simulink model "Test7"  (R2021a)
settings: Solver=FixedStepDiscrete  StartTime=0.0  StopTime=tsim  FixedStep=Ts  RelTol=1e-3  EnableMultiTasking=on
InitFcn:
  | Fs = 2048; Ts = 1/Fs;tsim = inf;
undefined symbols (not defined in the file or in its folder): DiscIntNeverNeededParam
libraries: sperte_lib x26, simulink x5, Quintic_Polynomial_Trajectory_Library x3, raspberrypiCommlib x2
(part 1 of 2)
settings Model: SimulationMode=external  Creator=20174295  LastModifiedBy=20212540
settings SolverCC: AlgebraicLoopSolver=TrustRegion  PositivePriorityOrder=on
settings DataIOCC: SaveOutput=off  DSMLogging=off  SaveTime=off  ReturnWorkspaceOutputs=off
settings OptimizationCC: EnhancedBackFolding=on  PassReuseOutputArgsThreshold=0  MaxStackSize=64  OptimizeBlockOrder=speed  DifferentSizesBufferReuse=on  OptimizationCustomize=off
settings DebuggingCC: InheritedTsInSrcMsg=none  ParameterTunabilityLossMsg=error  SFMachineParentedDataDiag=warning
settings HardwareCC: ProdBitPerPointer=32  ProdBitPerSizeT=32  ProdBitPerPtrDiffT=32  ProdLargestAtomicInteger=Long  ProdLargestAtomicFloat=Double  ProdWordSize=32  ProdLongLongMode=on  ProdHWDeviceType=ARM Compatible->ARM Cortex  UseEmbeddedCoderFeatures=off
settings RTWCC: SystemTargetFile=ert.tlc  HardwareBoard=Raspberry Pi  TLCOptions="-aInlineSetEventsForThisBaseRateFcn=TLC_FALSE -aSuppressMultiTaskScheduler=TLC_FALSE  -aRateBasedStepFcn=0"  TemplateMakefile=ert_default_tmf  PostCodeGenCommand="if (~verLessThan(\"matlab\", \"9.11\")) codertarget.postCodeGenHookCommand(h);  SPERTE_postGenFunc(modelName, buildInfo); else; SPERTE_postGenFunc(h, buildInfo); end"  Toolchain=GNU GCC Embedded Linux  BuildConfiguration=Faster Runs
settings CodeAppCC: ForceParamTrailComments=on  OperatorAnnotations=on
settings ERTTargetCC: ERTCustomFileBanners=off  SupportContinuousTime=on  SupportNonInlinedSFcns=on  RemoveResetFunc=off  SupportVariableSizeSignals=on  ModelStepFunctionPrototypeControlCompliant=off  ExtMode=on  ExtModeStaticAlloc=on  ExtModeMexArgs='10.55.0.1' 0 17726  ERTSrcFileBannerTemplate=codertarget_code_template.cgt  ERTHdrFileBannerTemplate=codertarget_code_template.cgt  ERTDataSrcFileTemplate=codertarget_code_template.cgt  ERTDataHdrFileTemplate=codertarget_code_template.cgt

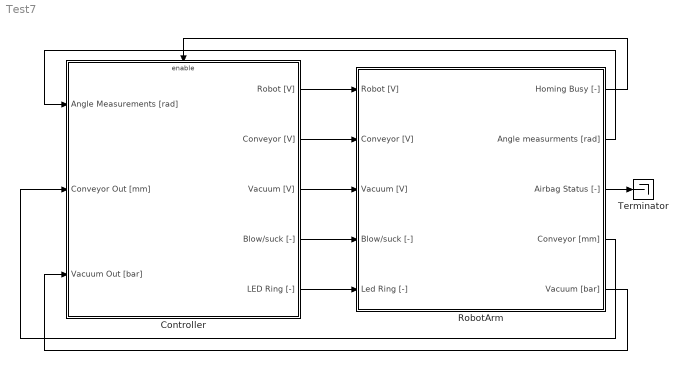
== system Test7 ==
  Controller : Subsystem
  RobotArm : Subsystem
      mask help:
      | Robot Arm
      | Hardware: Brom Mechatronica
      | Software: Victor Dolk, Quinten Swaan, Hugo Thelosen
      mask Display:
      | image(imread('picture_robot.jpg'))
      | color('red');port_label('output', 1, 'Homing Busy [-]')
      | port_label('output', 2, 'Angle Measurements [rad]')
      | port_label('output', 3, 'Airbag Status [-]')
      | port_label('input', 1, 'Input Robot [V]')
      | port_label('output', 4, 'Conveyor Belt [mm]')
      | port_label('output', 5, 'Vacuum Sensor [bar]')
      | port_label('input',2,'Input Conv [V]' )
      | port_label('input',3,'Input Vac [V]' )
      | port_label('input',4,'IO Vac [-]' )
      | port_label('input',5,'LED-Ring [-]' )
  Terminator : Terminator
  wires:
  RobotArm/4(Conveyor [mm]) -> Controller/2(Conveyor Out [mm])
  Controller/5(LED Ring [-]) -> RobotArm/5(Led Ring [-])
  Controller/1(Robot [V]) -> RobotArm/1(Robot [V])
  Controller/4(Blow/suck [-]) -> RobotArm/4(Blow/suck [-])
  RobotArm/1(Homing Busy [-]) -> Controller/Enable
  Controller/3("Vacuum [V] ") -> RobotArm/3(Vacuum [V])
  Controller/2("Conveyor [V] ") -> RobotArm/2(Conveyor [V])
  RobotArm/5(Vacuum [bar]) -> Controller/3(Vacuum Out [bar])
  RobotArm/3(Airbag Status [-]) -> Terminator/1
  RobotArm/2(Angle measurments [rad]) -> Controller/1(Angle Measurements [rad])

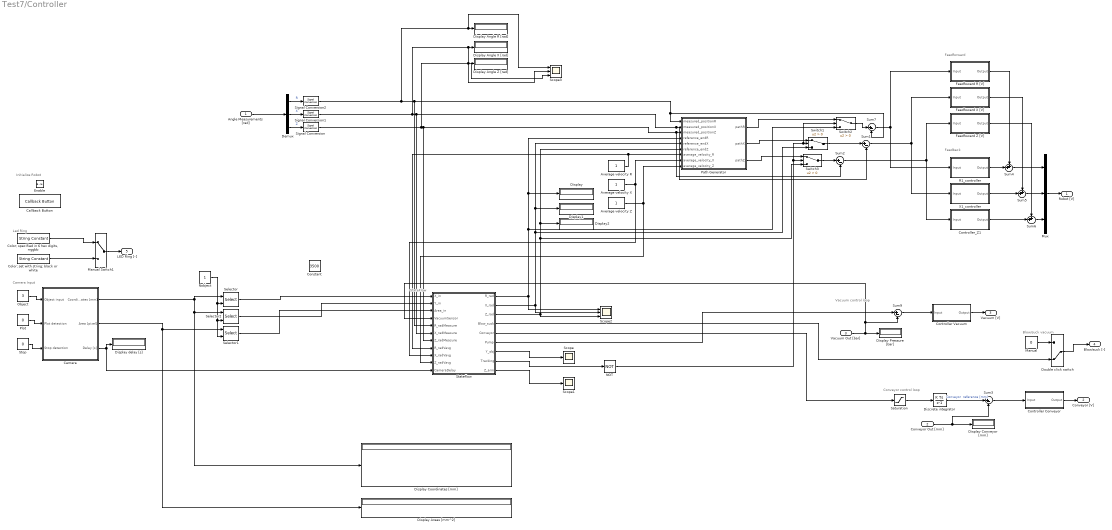
== system Test7/Controller ==
  note: Feedforward
  note: StateFlow
  note: Camera Input
  note: Vacuum control loop
  note: Conveyor control loop
  note: Blow/suck vacuum
  note: Led Ring
  note: Feedback
  note: Initialize Robot
  Angle Measurements [rad] : Inport
  Conveyor Out [mm] : Inport  Port=2
  Vacuum Out [bar] : Inport  Port=3
  "Enable " : EnablePort
  Average velocity R : Constant
  Average velocity X : Constant
  Average velocity Z : Constant
  Callback Button : CallbackButton  ButtonText=INITIALIZE MODEL
      settings: ClickFcn=|
      | robot_number = input('What is your Robot number?: ');
      | file_name_simulink = get_param(bdroot, 'Name');
      | load('calibration_matrix.mat');
      | [camera_calibration_x_pixels,camera_calibration_y_pixels,camera_calibration_pixels_per_mm,camera_calibration_ROI,robot_calibration_r,robot_calibration_x, robot_calibration_z] = Calibrate_Robot_Settings(robot_number,calibration)
      | 
      | set_param(file_name_simulink+"/RobotArm/Supervisor/set_robot_calibration_r",'Value',num2str(robot_calibration_r));
      | set_param(file_name_simulink+"/RobotArm/Supervisor/set_robot_calibration_x",'Value',num2str(robot_calibration_x));
      | set_param(file_name_simulink+"/RobotArm/Supervisor/set_robot_calibration_z",'Value',num2str(robot_calibration_z));
      | 
      | clear calibration
      | msgbox('Successfully initialized the model.');
  Camera : Subsystem
  Color; set with string; black or white : StringConstant  String='white'
  "Color; specified in 6 hex digits, rrggbb" : StringConstant  String='FF0000'
  Constant : Constant  Value=3500
  Controller Conveyor : Subsystem
  Controller Vacuum : Subsystem
  Controller_Z1 : Subsystem
  Demux : Demux  Outputs=3
  Discrete integrator : DiscreteIntegrator  SampleTime=-1  ICPrevOutput=DiscIntNeverNeededParam  ICPrevScaledInput=DiscIntNeverNeededParam
  Display : Display
  Display Angle R [rad] : Display
  Display Angle X [rad] : Display
  Display Angle Z [rad] : Display
  Display Areas [mm^2] : Display
  Display Conveyor [mm] : Display
  Display Coordinates [mm] : Display
  Display Pressure [bar] : Display
  Display delay [s] : Display
  Display1 : Display
  Display2 : Display
  Double click switch : ManualSwitch  CurrentSetting=0
  Feedfoward R [V] : Subsystem
  Feedfoward X [V] : Subsystem
  Feedfoward Z [V] : Subsystem
  Manual : Constant  Value=0
  Manual Switch1 : ManualSwitch
  Mux : Mux  Inputs=3
  NOT : Logic  Operator=NOT  IconShape=distinctive  AllPortsSameDT=off  OutDataTypeStr=boolean
  Nobject : Constant
  Object : Constant  Value=3
  Path Generator : Subsystem
  Plot : Constant  Value=0
  R1_controller : Subsystem
  "Saturation " : Saturate  UpperLimit=100  LowerLimit=-100
  Scope : Scope
  Scope1 : Scope
  Scope2 : Scope  NumInputPorts=3
  Scope3 : Scope  NumInputPorts=3
  Selector : Selector  NumberOfDimensions=2  InputPortWidth=3  IndexOptions=Index vector (dialog),Index vector (port)  Indices=1,1  OutputSizes=1,1
  Selector1 : Selector  InputPortWidth=3  IndexOptions=Index vector (port)  Indices=[1 3]  OutputSizes=1
  Selector2 : Selector  NumberOfDimensions=2  InputPortWidth=3  IndexOptions=Index vector (dialog),Index vector (port)  Indices=2,1  OutputSizes=1,1
  Signal Conversion : SignalConversion  OverrideOpt=off
  Signal Conversion1 : SignalConversion  OverrideOpt=off
  Signal Conversion2 : SignalConversion  OverrideOpt=off
  "Stateflow " : Stateflow chart  TreatAsAtomicUnit=on
  Stop : Constant  Value=0
  Sum1 : Sum  Inputs=|+-  InputSameDT=on  SaturateOnIntegerOverflow=on  OutDataTypeStr=Inherit: Same as first input
  Sum2 : Sum  Inputs=|+-  InputSameDT=on  SaturateOnIntegerOverflow=on  OutDataTypeStr=Inherit: Same as first input
  Sum3 : Sum  Inputs=|+-
  Sum4 : Sum  Inputs=++|  InputSameDT=on  SaturateOnIntegerOverflow=on  OutDataTypeStr=Inherit: Same as first input
  Sum5 : Sum  Inputs=++|  InputSameDT=on  SaturateOnIntegerOverflow=on  OutDataTypeStr=Inherit: Same as first input
  Sum6 : Sum  Inputs=++|  InputSameDT=on  SaturateOnIntegerOverflow=on  OutDataTypeStr=Inherit: Same as first input
  Sum7 : Sum  Inputs=|+-  InputSameDT=on  SaturateOnIntegerOverflow=on  OutDataTypeStr=Inherit: Same as first input
  Sum9 : Sum  Inputs=|+-
  Switch1 : Switch  Criteria=u2 > Threshold
  Switch2 : Switch  Criteria=u2 > Threshold
  Switch3 : Switch  Criteria=u2 > Threshold
  X1_controller : Subsystem
  Robot [V] : Outport
  "Conveyor [V] " : Outport  Port=2
  "Vacuum [V] " : Outport  Port=3
  Blow/suck [-] : Outport  Port=4
  LED Ring [-] : Outport  Port=5
  wires:
  Sum5/1 -> Mux/2
  Sum4/1 -> Mux/1
  Demux/3 -> Signal Conversion/1  "Z"
  Signal Conversion1/1 -> "Stateflow "/6(X_radMeasure), Path Generator/2(measured_positionX), Sum1/2, Scope3/2, Display Angle X [rad]/1
  Angle Measurements [rad]/1 -> Demux/1
  Demux/1 -> Signal Conversion2/1  "R"
  Mux/1 -> Robot [V]/1
  Signal Conversion/1 -> "Stateflow "/7(Z_radMeasure), Path Generator/3(measured_positionZ), Sum2/2, Scope3/3, Display Angle Z [rad]/1
  Sum6/1 -> Mux/3
  Demux/2 -> Signal Conversion1/1  "X"
  Signal Conversion2/1 -> "Stateflow "/5(R_radMeasure), Sum7/2, Path Generator/1(measured_positionR), Scope3/1, Display Angle R [rad]/1
  Manual Switch1/1 -> LED Ring [-]/1
  Conveyor Out [mm]/1 -> Sum3/2, Display Conveyor [mm]/1
  Color; set with string; black or white/1 -> Manual Switch1/2
  "Color; specified in 6 hex digits, rrggbb"/1 -> Manual Switch1/1
  Camera/1(Coordinates [mm]) -> Selector/1, Display Coordinates [mm]/1, Selector2/1
  Controller Vacuum/1(Output) -> "Vacuum [V] "/1
  Sum9/1 -> Controller Vacuum/1(Input)
  Vacuum Out [bar]/1 -> Sum9/2, "Stateflow "/4(VacuumSensor), Display Pressure [bar]/1
  Camera/2(Area [pixel]) -> Display Areas [mm^2]/1, Selector1/1
  Camera/3(Delay [s]) -> Display delay [s]/1, "Stateflow "/11(CameraDelay)
  Manual/1 -> Double click switch/1
  Plot/1 -> Camera/2(Plot detection)
  Object/1 -> Camera/1(Object input)
  Stop/1 -> Camera/3(Stop detection)
  Double click switch/1 -> Blow/suck [-]/1
  "Saturation "/1 -> Discrete integrator/1
  Discrete integrator/1 -> Sum3/1  "Conveyor  reference [mm]"
  Sum3/1 -> Controller Conveyor/1(Input)
  Controller Conveyor/1(Output) -> "Conveyor [V] "/1
  Feedfoward R [V]/1(Output) -> Sum4/1
  "Stateflow "/5(Conveyor) -> "Saturation "/1
  "Stateflow "/4(Blow_suck) -> Double click switch/2
  Nobject/1 -> Selector1/2, Selector2/2, Selector/2
  Selector1/1 -> "Stateflow "/3(Area_in)
  Sum7/1 -> R1_controller/1(Input), Feedfoward R [V]/1(Input)
  Sum1/1 -> X1_controller/1(Input), Feedfoward X [V]/1(Input)
  Sum2/1 -> Feedfoward Z [V]/1(Input), Controller_Z1/1(Input)
  Feedfoward X [V]/1(Output) -> Sum5/1
  Feedfoward Z [V]/1(Output) -> Sum6/1
  Average velocity R/1 -> Path Generator/7(average_velocity_R), "Stateflow "/8(R_radVavg)
  Average velocity X/1 -> Path Generator/8(average_velocity_X), "Stateflow "/9(X_radVavg)
  Average velocity Z/1 -> "Stateflow "/10(Z_radVavg), Path Generator/9(average_velocity_Z)
  "Stateflow "/6(Pump) -> Sum9/1
  R1_controller/1(Output) -> Sum4/2
  X1_controller/1(Output) -> Sum5/2
  Controller_Z1/1(Output) -> Sum6/2
  Selector2/1 -> "Stateflow "/2(Y_in)
  Path Generator/2(pathX) -> Switch1/1
  Path Generator/3(pathZ) -> Switch3/1
  "Stateflow "/1(R_rad) -> Scope2/1, Path Generator/4(reference_endR), Display/1, Switch2/3
  "Stateflow "/2(X_rad) -> Scope2/2, Display1/1, Path Generator/5(reference_endX), Switch1/3
  "Stateflow "/3(Z_rad) -> Scope2/3, Display2/1, Path Generator/6(reference_endZ), Switch3/3
  Path Generator/1(pathR) -> Switch2/1
  "Stateflow "/7(Y_obj) -> Scope/1
  Selector/1 -> "Stateflow "/1(X_in)
  Switch2/1 -> Sum7/1
  Switch1/1 -> Sum1/1
  Switch3/1 -> Sum2/1
  NOT/1 -> Switch3/2, Switch2/2, Switch1/2
  "Stateflow "/8(Tracking) -> NOT/1
  "Stateflow "/9(Z_arm) -> Scope1/1

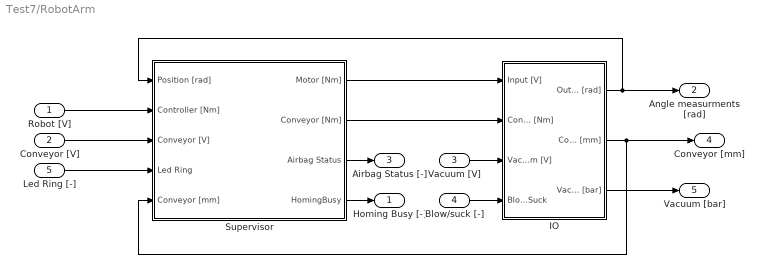
== system Test7/RobotArm ==
  Robot [V] : Inport
  Conveyor [V] : Inport  Port=2
  Vacuum [V] : Inport  Port=3
  Blow/suck [-] : Inport  Port=4
  Led Ring [-] : Inport  Port=5
  IO : Subsystem
  Supervisor : Subsystem
  Homing Busy [-] : Outport
  Angle measurments [rad] : Outport  Port=2
  Airbag Status [-] : Outport  Port=3
  Conveyor [mm] : Outport  Port=4
  Vacuum [bar] : Outport  Port=5
  wires:
  Robot [V]/1 -> Supervisor/2(Controller [Nm])
  IO/1(Output [rad]) -> Supervisor/1(Position [rad]), Angle measurments [rad]/1
  Supervisor/4(HomingBusy) -> Homing Busy [-]/1
  Supervisor/3(Airbag Status) -> Airbag Status [-]/1
  Supervisor/1(Motor [Nm]) -> IO/1(Input [V])
  IO/3(Vacuum [bar]) -> Vacuum [bar]/1
  Conveyor [V]/1 -> Supervisor/3(Conveyor [V])
  Vacuum [V]/1 -> IO/3(Vacuum [V])
  Supervisor/2(Conveyor [Nm]) -> IO/2(Conveyor [Nm])
  Blow/suck [-]/1 -> IO/4(Blow_Suck)
  IO/2(Conveyor [mm]) -> Supervisor/5(Conveyor [mm]), Conveyor [mm]/1
  Led Ring [-]/1 -> Supervisor/4(Led Ring)

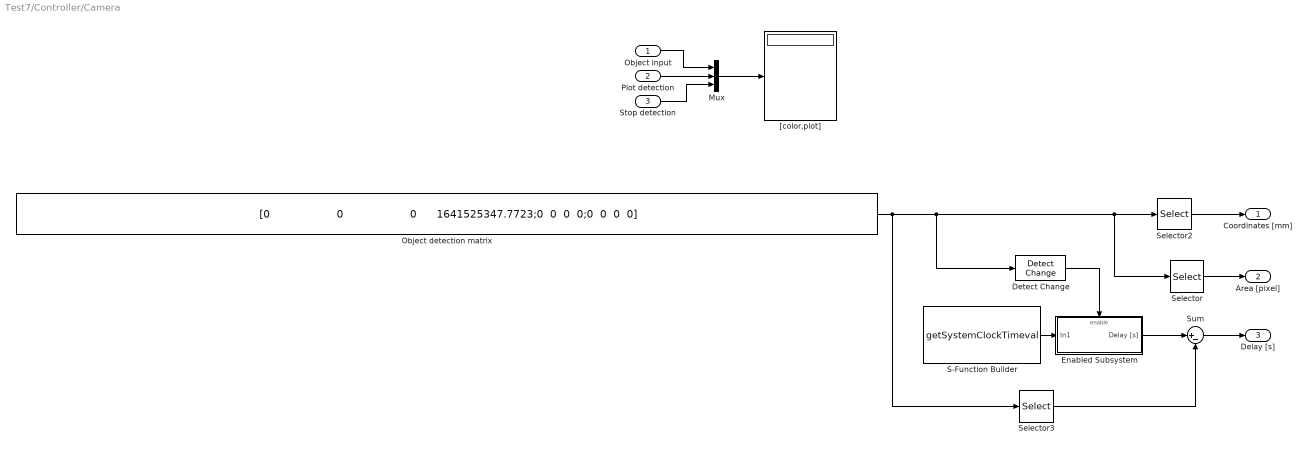
== system Test7/Controller/Camera ==
  Object input : Inport
  Plot detection : Inport  Port=2
  Stop detection : Inport  Port=3
  Detect Change : simulink/Logic and Bit Operations/Detect Change  vinit=0  OutDataTypeStr=boolean
  Enabled Subsystem : Subsystem  TreatAsAtomicUnit=on
  Mux : Mux  Inputs=3
  Object detection matrix : Constant  Value="[0                    0                    0      1641525347.7723;0  0  0  0;0  0  0  0]"  VectorParams1D=off
  S-Function Builder : S-Function  InitFcn=try, set_param(gcb,'FunctionName','getSystemClockTimeval'), end  FunctionName=getSystemClockTimeval  SFunctionModules=getSystemClockTimeval_wrapper  SFunctionDeploymentMode=off  EnableBusSupport=off  mask(S-Function Builder){}
      mask help: Simulink:masks:SFunctionBuilder_MD
      mask init:
      | val = [[.9  0.75 0.75 1 1 .9 .9 1]',[1 1 0.75 0.75 .9 .9 1 .9]'];try , sys = get_param(gcb,'SfunBuilderFcnName');if isempty(sys), sys = get_param(gcb,'FunctionName'); end,catch, sys = get_param(gcb,'FunctionName'); end
      settings: CopyFcn=set_param(gcbh,'LinkStatus','none')  PreSaveFcn=try, set_param(gcb,'FunctionName','getSystemClockTimeval'), end  OpenFcn=sfunctionwizard(gcbh)
      mask Display: plot(val(:,1),val(:,2)),disp(sys),port_label('output',1,'y2')
  Selector : Selector  NumberOfDimensions=2  InputPortWidth=3  IndexOptions=Index vector (dialog),Index vector (dialog)  Indices=[3],[1:3]  OutputSizes=1,1
  Selector2 : Selector  NumberOfDimensions=2  InputPortWidth=3  IndexOptions=Index vector (dialog),Index vector (dialog)  Indices=[1:2],[1:3]  OutputSizes=1,1
  Selector3 : Selector  NumberOfDimensions=2  InputPortWidth=3  IndexOptions=Index vector (dialog),Index vector (dialog)  Indices=1,4  OutputSizes=1,1
  Sum : Sum  Inputs=|+-
  "[color,plot]" : Display
  Coordinates [mm] : Outport
  Area [pixel] : Outport  Port=2
  Delay [s] : Outport  Port=3
  wires:
  Object input/1 -> Mux/1
  Plot detection/1 -> Mux/2
  Mux/1 -> "[color,plot]"/1
  Stop detection/1 -> Mux/3
  Selector2/1 -> Coordinates [mm]/1
  Object detection matrix/1 -> Selector3/1, Detect Change/1, Selector/1, Selector2/1
  Detect Change/1 -> Enabled Subsystem/Enable
  S-Function Builder/1 -> Enabled Subsystem/1(In1)
  Enabled Subsystem/1(Delay [s]) -> Sum/1
  Sum/1 -> Delay [s]/1
  Selector3/1 -> Sum/2
  Selector/1 -> Area [pixel]/1

== system Test7/Controller/Controller Conveyor ==
  Input : Inport
  Dct1lowpass : sperte_lib/Dct1lowpass  f_den=30
      settings: SourceProductName=SPERTE project library
  Dctintegrator3 : S-Function  FunctionName=dweakint  Parameters=f_num, 0.001  SFunctionDeploymentMode=off  EnableBusSupport=off  mask(dctools){f_num=0}
      mask prompts: f_num "Zero [Hz]"
      mask help: This block implements a discrete time weak integrator filter.
      mask Display: disp('DCT integrator')
  Dctleadlag : sperte_lib/Dctleadlag  f_num=3  f_den=20
      settings: SourceProductName=SPERTE project library
  Gain1 : Gain  Gain=10*2.5/500
  Output : Outport
  wires:
  Input/1 -> Gain1/1
  Dctintegrator3/1 -> Dct1lowpass/1
  Dctleadlag/1 -> Output/1
  Gain1/1 -> Dctintegrator3/1
  Dct1lowpass/1 -> Dctleadlag/1

== system Test7/Controller/Controller Vacuum ==
  Input : Inport
  Gain1 : Gain  Gain=-10
  Output : Outport
  wires:
  Input/1 -> Gain1/1
  Gain1/1 -> Output/1

== system Test7/Controller/Controller_Z1 ==
  Input : Inport
  Dct1lowpass1 : sperte_lib/Dct1lowpass  f_den=200
      settings: SourceProductName=SPERTE project library
  Dctintegrator2 : S-Function  FunctionName=dweakint  Parameters=f_num, 0.001  SFunctionDeploymentMode=off  EnableBusSupport=off  mask(dctools){f_num=1.7}
      mask prompts: f_num "Zero [Hz]"
      mask help: This block implements a discrete time weak integrator filter.
      mask Display: disp('DCT integrator')
  Dctleadlag3 : S-Function  FunctionName=dleadlag  Parameters=f_num, f_den, 0.001  SFunctionDeploymentMode=off  EnableBusSupport=off  mask(dctools){f_num=7, f_den=75}
      mask prompts: f_num "Zero [Hz]"; f_den "Pole [Hz]"
      mask help: This block implements a discrete time leadlag filter.
      mask Display: disp('DCT leadlag')
  Gain2 : Gain  Gain=25
  Output : Outport
  wires:
  Input/1 -> Gain2/1
  Dctintegrator2/1 -> Dctleadlag3/1
  Gain2/1 -> Dctintegrator2/1
  Dctleadlag3/1 -> Dct1lowpass1/1
  Dct1lowpass1/1 -> Output/1

== system Test7/Controller/Feedfoward R [V] ==
  Input : Inport
  Derivative : Derivative
  Derivative1 : Derivative
  Gain1 : Gain  Gain=0
  Gain2 : Gain  Gain=0
  Inertia compensation : Gain  Gain=0
  Sign : Signum
  Sum : Sum  Inputs=+++
  Output : Outport
  wires:
  Input/1 -> Derivative/1
  Derivative/1 -> Sign/1, Gain1/1, Derivative1/1
  Sum/1 -> Output/1
  Gain2/1 -> Sum/1
  Gain1/1 -> Sum/2
  Inertia compensation/1 -> Sum/3
  Derivative1/1 -> Inertia compensation/1
  Sign/1 -> Gain2/1

== system Test7/Controller/Feedfoward X [V] ==
  Input : Inport
  Derivative : Derivative
  Derivative1 : Derivative
  Gain1 : Gain  Gain=0
  Gain2 : Gain  Gain=0
  Inertia compensation : Gain  Gain=0
  Sign : Signum
  Sum : Sum  Inputs=+++
  Output : Outport
  wires:
  Sign/1 -> Gain2/1
  Sum/1 -> Output/1
  Gain1/1 -> Sum/2
  Gain2/1 -> Sum/1
  Derivative1/1 -> Inertia compensation/1
  Inertia compensation/1 -> Sum/3
  Derivative/1 -> Sign/1, Gain1/1, Derivative1/1
  Input/1 -> Derivative/1

== system Test7/Controller/Feedfoward Z [V] ==
  Input : Inport
  Derivative : Derivative
  Derivative1 : Derivative
  Gain1 : Gain  Gain=0
  Gain2 : Gain  Gain=0
  Inertia compensation : Gain  Gain=0
  Sign : Signum
  Sum : Sum  Inputs=+++
  Output : Outport
  wires:
  Sign/1 -> Gain2/1
  Sum/1 -> Output/1
  Gain1/1 -> Sum/2
  Gain2/1 -> Sum/1
  Derivative1/1 -> Inertia compensation/1
  Inertia compensation/1 -> Sum/3
  Derivative/1 -> Sign/1, Gain1/1, Derivative1/1
  Input/1 -> Derivative/1

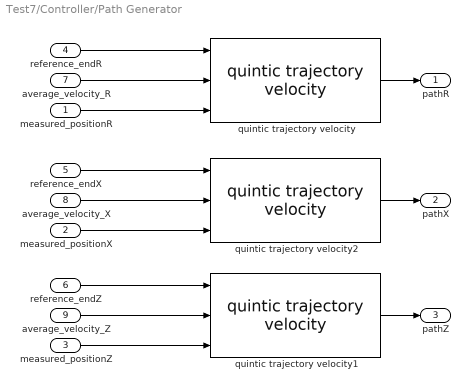
== system Test7/Controller/Path Generator ==
  measured_positionR : Inport
  measured_positionX : Inport  Port=2
  measured_positionZ : Inport  Port=3
  reference_endR : Inport  Port=4
  reference_endX : Inport  Port=5
  reference_endZ : Inport  Port=6
  average_velocity_R : Inport  Port=7
  average_velocity_X : Inport  Port=8
  average_velocity_Z : Inport  Port=9
  quintic trajectory velocity : Quintic_Polynomial_Trajectory_Library/quintic trajectory velocity  SystemSampleTime=-1  VariantActivationTime=update diagram  Latency=0  AutoFrameSizeCalculation=off
      settings: SourceProductName=Robotarm library
  quintic trajectory velocity1 : Quintic_Polynomial_Trajectory_Library/quintic trajectory velocity  SystemSampleTime=-1  VariantActivationTime=update diagram  Latency=0  AutoFrameSizeCalculation=off
      settings: SourceProductName=Robotarm library
  quintic trajectory velocity2 : Quintic_Polynomial_Trajectory_Library/quintic trajectory velocity  SystemSampleTime=-1  VariantActivationTime=update diagram  Latency=0  AutoFrameSizeCalculation=off
      settings: SourceProductName=Robotarm library
  pathR : Outport
  pathX : Outport  Port=2
  pathZ : Outport  Port=3
  wires:
  reference_endR/1 -> quintic trajectory velocity/1
  measured_positionR/1 -> quintic trajectory velocity/3
  average_velocity_R/1 -> quintic trajectory velocity/2
  average_velocity_X/1 -> quintic trajectory velocity2/2
  average_velocity_Z/1 -> quintic trajectory velocity1/2
  measured_positionX/1 -> quintic trajectory velocity2/3
  measured_positionZ/1 -> quintic trajectory velocity1/3
  reference_endX/1 -> quintic trajectory velocity2/1
  reference_endZ/1 -> quintic trajectory velocity1/1
  quintic trajectory velocity/1 -> pathR/1
  quintic trajectory velocity2/1 -> pathX/1
  quintic trajectory velocity1/1 -> pathZ/1

== system Test7/Controller/R1_controller ==
  Input : Inport
  Dct1lowpass1 : sperte_lib/Dct1lowpass  f_den=100
      settings: SourceProductName=SPERTE project library
  Dctintegrator2 : S-Function  FunctionName=dweakint  Parameters=f_num, 0.001  SFunctionDeploymentMode=off  EnableBusSupport=off  mask(dctools){f_num=1.35}
      mask prompts: f_num "Zero [Hz]"
      mask help: This block implements a discrete time weak integrator filter.
      mask Display: disp('DCT integrator')
  Dctleadlag3 : S-Function  FunctionName=dleadlag  Parameters=f_num, f_den, 0.001  SFunctionDeploymentMode=off  EnableBusSupport=off  mask(dctools){f_num=8, f_den=75}
      mask prompts: f_num "Zero [Hz]"; f_den "Pole [Hz]"
      mask help: This block implements a discrete time leadlag filter.
      mask Display: disp('DCT leadlag')
  Gain1 : Gain  Gain=40
  Output : Outport
  wires:
  Gain1/1 -> Dctintegrator2/1
  Dctintegrator2/1 -> Dctleadlag3/1
  Input/1 -> Gain1/1
  Dctleadlag3/1 -> Dct1lowpass1/1
  Dct1lowpass1/1 -> Output/1

== system Test7/Controller/X1_controller ==
  Input : Inport
  Dct1lowpass1 : sperte_lib/Dct1lowpass  f_den=200
      settings: SourceProductName=SPERTE project library
  Dctintegrator2 : S-Function  FunctionName=dweakint  Parameters=f_num, 0.001  SFunctionDeploymentMode=off  EnableBusSupport=off  mask(dctools){f_num=2}
      mask prompts: f_num "Zero [Hz]"
      mask help: This block implements a discrete time weak integrator filter.
      mask Display: disp('DCT integrator')
  Dctleadlag3 : S-Function  FunctionName=dleadlag  Parameters=f_num, f_den, 0.001  SFunctionDeploymentMode=off  EnableBusSupport=off  mask(dctools){f_num=10, f_den=70}
      mask prompts: f_num "Zero [Hz]"; f_den "Pole [Hz]"
      mask help: This block implements a discrete time leadlag filter.
      mask Display: disp('DCT leadlag')
  Gain2 : Gain  Gain=17
  Output : Outport
  wires:
  Input/1 -> Gain2/1
  Dctintegrator2/1 -> Dctleadlag3/1
  Gain2/1 -> Dctintegrator2/1
  Dctleadlag3/1 -> Dct1lowpass1/1
  Dct1lowpass1/1 -> Output/1

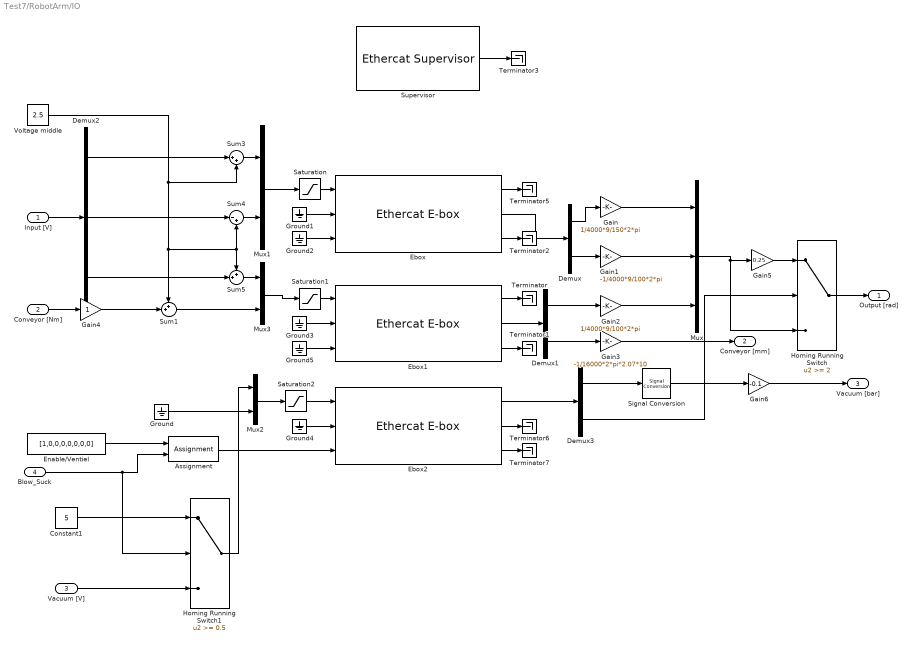
== system Test7/RobotArm/IO ==
  Input [V] : Inport
  Conveyor [Nm] : Inport  Port=2
  Vacuum [V] : Inport  Port=3
  Blow_Suck : Inport  Port=4
  Assignment : Assignment  DiagnosticForDimensions=Warning  IndexOptions=Index vector (dialog)  Indices=2  OutputSizes=1
  Constant1 : Constant  Value=5
  Demux : Demux  Outputs=2
  Demux1 : Demux  Outputs=2
  Demux2 : Demux  Outputs=3
  Demux3 : Demux  Outputs=2
  Ebox : sperte_lib/Ethercat E-box  Priority=-2  link_id=0
      settings: SourceProductName=SPERTE project library
  Ebox1 : sperte_lib/Ethercat E-box  Priority=-2  link_id=1
      settings: SourceProductName=SPERTE project library
  Ebox2 : sperte_lib/Ethercat E-box  Priority=-2  link_id=2
      settings: SourceProductName=SPERTE project library
  Enable/Ventiel : Constant  Value=[1,0,0,0,0,0,0,0]
  Gain : Gain  Gain=1/4000*9/150*2*pi
  Gain1 : Gain  Gain=-1/4000*9/100*2*pi
  Gain2 : Gain  Gain=1/4000*9/100*2*pi
  Gain3 : Gain  Gain=-1/16000*2*pi*2.07*10
  Gain4 : Gain
  Gain5 : Gain  Gain=0.25
  Gain6 : Gain  Gain=-0.1
  Ground{,1..5} (6 alike) : Ground
  Homing Running Switch : Switch  Threshold=2
  Homing Running Switch1 : Switch  Threshold=0.5
  Mux : Mux  Inputs=3
  Mux1 : Mux  Inputs=2
  Mux2 : Mux  Inputs=2
  Mux3 : Mux  Inputs=2
  Saturation : Saturate  UpperLimit=5  LowerLimit=0
  Saturation1 : Saturate  UpperLimit=5  LowerLimit=0
  Saturation2 : Saturate  UpperLimit=5  LowerLimit=0
  Signal Conversion : SignalConversion  OverrideOpt=off
  Sum1 : Sum  Inputs=++|
  Sum3 : Sum  Inputs=|++
  Sum4 : Sum  Inputs=|-+
  Sum5 : Sum  Inputs=++|
  Supervisor : sperte_lib/Ethercat Supervisor  Description=Must be executed first, keep at -1 priority (highest)  Priority=-3  portid=0  ectimeout=500
      settings: SourceProductName=SPERTE project library
  Terminator{,1..3,5..7} (7 alike) : Terminator
  Voltage middle : Constant  Value=2.5
  Output [rad] : Outport
  Conveyor [mm] : Outport  Port=2
  Vacuum [bar] : Outport  Port=3
  wires:
  Demux1/2 -> Gain3/1
  Ground1/1 -> Ebox/2
  Demux/2 -> Gain1/1
  Mux3/1 -> Saturation1/1
  Demux2/2 -> Sum4/1
  Sum5/1 -> Mux3/1
  Saturation/1 -> Ebox/1
  Ebox/3 -> Terminator2/1
  Saturation1/1 -> Ebox1/1
  Mux1/1 -> Saturation/1
  Gain1/1 -> Mux/2
  Sum3/1 -> Mux1/1
  Voltage middle/1 -> Sum4/2, Sum5/1, Sum1/1, Sum3/2
  Ground3/1 -> Ebox1/2
  Gain2/1 -> Mux/3
  Gain/1 -> Mux/1
  Demux2/1 -> Sum3/1
  Ebox1/2 -> Demux1/1
  Ground2/1 -> Ebox/3
  Ebox/2 -> Demux/1
  Sum4/1 -> Mux1/2
  Demux/1 -> Gain/1
  Demux1/1 -> Gain2/1
  Ebox1/3 -> Terminator1/1
  Input [V]/1 -> Demux2/1
  Demux2/3 -> Sum5/2
  Supervisor/1 -> Terminator3/1
  Gain3/1 -> Conveyor [mm]/1
  Ebox2/2 -> Terminator6/1
  Ebox2/3 -> Terminator7/1
  Ground4/1 -> Ebox2/2
  Assignment/1 -> Ebox2/3
  Enable/Ventiel/1 -> Assignment/1
  Blow_Suck/1 -> Homing Running Switch1/2, Assignment/2
  Sum1/1 -> Mux3/2
  Mux2/1 -> Saturation2/1
  Vacuum [V]/1 -> Homing Running Switch1/3
  Ground/1 -> Mux2/2
  Saturation2/1 -> Ebox2/1
  Demux3/2 -> Homing Running Switch/2
  Demux3/1 -> Signal Conversion/1
  Ebox1/1 -> Terminator/1
  Ebox/1 -> Terminator5/1
  Ebox2/1 -> Demux3/1
  Ground5/1 -> Ebox1/3
  Gain4/1 -> Sum1/2
  Conveyor [Nm]/1 -> Gain4/1
  Homing Running Switch/1 -> Output [rad]/1
  Mux/1 -> Homing Running Switch/3, Gain5/1
  Gain5/1 -> Homing Running Switch/1
  Signal Conversion/1 -> Gain6/1
  Gain6/1 -> Vacuum [bar]/1
  Constant1/1 -> Homing Running Switch1/1
  Homing Running Switch1/1 -> Mux2/1

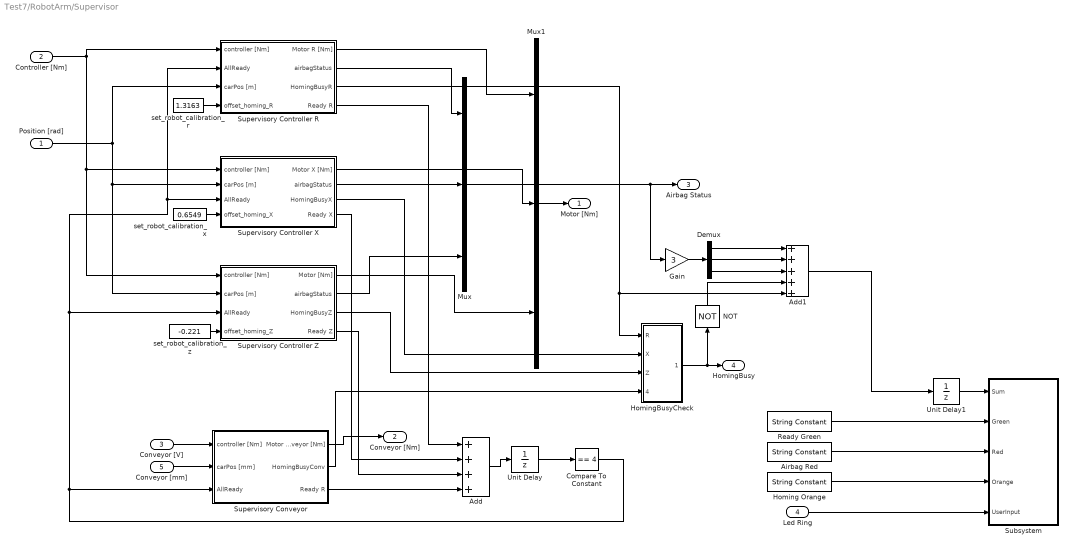
== system Test7/RobotArm/Supervisor ==
  Position [rad] : Inport
  Controller [Nm] : Inport  Port=2
  Conveyor [V] : Inport  Port=3
  Led Ring : Inport  Port=4
  Conveyor [mm] : Inport  Port=5
  Add : Sum  Inputs=++++
  Add1 : Sum  Inputs=+++++
  Airbag Red : StringConstant  String='00FF0000'
  Compare To Constant : simulink/Logic and Bit Operations/Compare To Constant  relop===  const=4  OutDataTypeStr=boolean
  Demux : Demux  Outputs=3
  Gain : Gain  Gain=3
  Homing Orange : StringConstant  String='00FF3900'
  HomingBusyCheck : Subsystem
  Mux : Mux  Inputs=3
  Mux1 : Mux  Inputs=3
  NOT : Logic  Operator=NOT  IconShape=distinctive  AllPortsSameDT=off  OutDataTypeStr=boolean
  Ready Green : StringConstant  String='0000FF00'
  Subsystem : Subsystem
  Supervisory Controller R : Subsystem
  Supervisory Controller X : Subsystem
  Supervisory Controller Z : Subsystem
  Supervisory Conveyor : Subsystem
  Unit Delay : UnitDelay  SampleTime=-1  HasFrameUpgradeWarning=on
  Unit Delay1 : UnitDelay  SampleTime=-1  HasFrameUpgradeWarning=on
  set_robot_calibration_r : Constant  Value=1.3163
  set_robot_calibration_x : Constant  Value=0.6549
  set_robot_calibration_z : Constant  Value=-0.221
  Motor [Nm] : Outport
  Conveyor [Nm] : Outport  Port=2
  Airbag Status : Outport  Port=3
  HomingBusy : Outport  Port=4
  wires:
  Controller [Nm]/1 -> Supervisory Controller R/1(controller [Nm]), Supervisory Controller Z/1(controller [Nm]), Supervisory Controller X/1(controller [Nm])
  Supervisory Controller R/2(airbagStatus) -> Mux/1
  Supervisory Controller X/2(airbagStatus) -> Mux/2
  Supervisory Controller Z/2(airbagStatus) -> Mux/3
  Supervisory Controller R/1(Motor R [Nm]) -> Mux1/1
  Supervisory Controller X/1(Motor X [Nm]) -> Mux1/2
  Supervisory Controller Z/1(Motor [Nm]) -> Mux1/3
  Position [rad]/1 -> Supervisory Controller R/3(carPos [m]), Supervisory Controller Z/2(carPos [m]), Supervisory Controller X/2(carPos [m])
  Mux1/1 -> Motor [Nm]/1
  Supervisory Controller R/3(HomingBusyR) -> HomingBusyCheck/1(R), Add1/5
  Supervisory Controller X/3(HomingBusyX) -> HomingBusyCheck/2(X)
  Supervisory Controller Z/3(HomingBusyZ) -> HomingBusyCheck/3(Z)
  HomingBusyCheck/1(Out1) -> NOT/1, HomingBusy/1
  Supervisory Controller R/4(Ready R) -> Add/1
  Supervisory Controller X/4(Ready X) -> Add/2
  Supervisory Controller Z/4(Ready Z) -> Add/3
  Compare To Constant/1 -> Supervisory Controller Z/3(AllReady), Supervisory Controller X/3(AllReady), Supervisory Controller R/2(AllReady), Supervisory Conveyor/3(AllReady)
  Add/1 -> Unit Delay/1
  Unit Delay/1 -> Compare To Constant/1
  Conveyor [V]/1 -> Supervisory Conveyor/1(controller [Nm])
  Supervisory Conveyor/3(Ready R) -> Add/4
  Supervisory Conveyor/1(Motor Conveyor [Nm]) -> Conveyor [Nm]/1
  Supervisory Conveyor/2(HomingBusyConv) -> HomingBusyCheck/4(Conv)
  set_robot_calibration_r/1 -> Supervisory Controller R/4(offset_homing_R)
  set_robot_calibration_x/1 -> Supervisory Controller X/4(offset_homing_X)
  set_robot_calibration_z/1 -> Supervisory Controller Z/4(offset_homing_Z)
  Conveyor [mm]/1 -> Supervisory Conveyor/2(carPos [mm])
  Mux/1 -> Gain/1, Airbag Status/1
  Demux/1 -> Add1/1
  Demux/2 -> Add1/2
  Demux/3 -> Add1/3
  NOT/1 -> Add1/4
  Gain/1 -> Demux/1
  Ready Green/1 -> Subsystem/2(Green)
  Add1/1 -> Unit Delay1/1
  Airbag Red/1 -> Subsystem/3(Red)
  Homing Orange/1 -> Subsystem/4(Orange)
  Led Ring/1 -> Subsystem/5(UserInput)
  Unit Delay1/1 -> Subsystem/1(Sum)

== system Test7/Controller/Camera/Enabled Subsystem ==
  In1 : Inport
  Enable : EnablePort
  Delay [s] : Outport
  wires:
  In1/1 -> Delay [s]/1

== system Test7/RobotArm/Supervisor/HomingBusyCheck ==
  R : Inport
  X : Inport  Port=2
  Z : Inport  Port=3
  Conv : Inport  Port=4
  Add : Sum  Inputs=++++
  Add1 : Sum  Inputs=+-
  Constant : Constant
  Sign : Signum
  Out1 : Outport
  wires:
  Add/1 -> Sign/1
  R/1 -> Add/1
  X/1 -> Add/2
  Z/1 -> Add/3
  Constant/1 -> Add1/1
  Sign/1 -> Add1/2
  Add1/1 -> Out1/1
  Conv/1 -> Add/4

== system Test7/RobotArm/Supervisor/Subsystem ==
  Sum : Inport
  Green : Inport  Port=2
  Red : Inport  Port=3
  Orange : Inport  Port=4
  UserInput : Inport  Port=5
  Homing Running Switch : Switch  Threshold=0.5
  Homing Running Switch1 : Switch  Threshold=2.5
  Homing Running Switch2 : Switch  Threshold=50
  LED Ring : Subsystem
  wires:
  Homing Running Switch/1 -> LED Ring/1(U)
  Green/1 -> Homing Running Switch2/1
  UserInput/1 -> Homing Running Switch/3
  Homing Running Switch1/1 -> Homing Running Switch/1
  Red/1 -> Homing Running Switch2/3
  Orange/1 -> Homing Running Switch1/3
  Sum/1 -> Homing Running Switch2/2, Homing Running Switch1/2, Homing Running Switch/2
  Homing Running Switch2/1 -> Homing Running Switch1/1

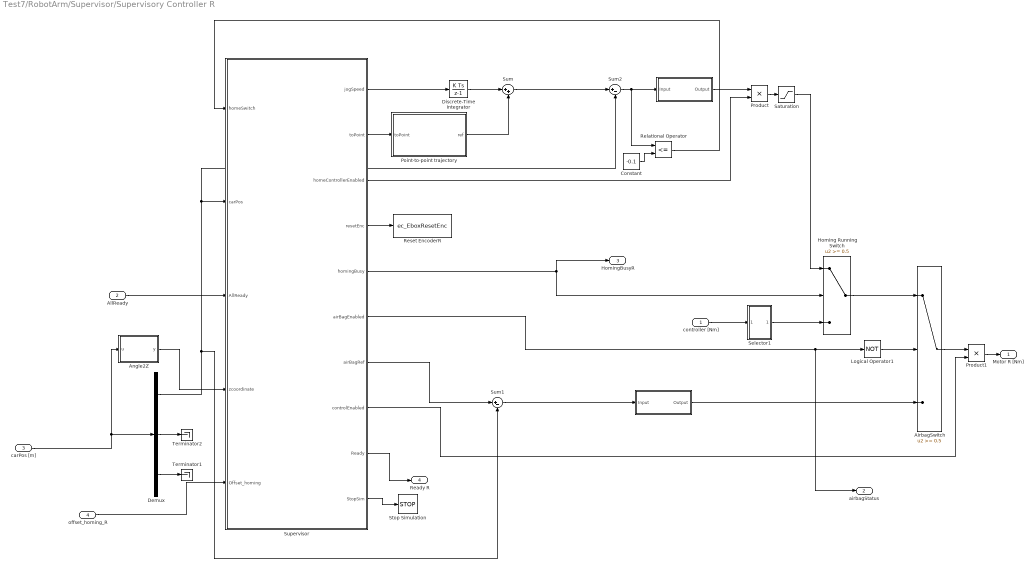
== system Test7/RobotArm/Supervisor/Supervisory Controller R ==
  controller [Nm] : Inport
  AllReady : Inport  Port=2
  carPos [m] : Inport  Port=3
  offset_homing_R : Inport  Port=4
  " " : Subsystem
  "   " : Subsystem
  AirbagSwitch : Switch  Threshold=0.5
  Angle2Z : MATLAB Function  TreatAsAtomicUnit=on
  Constant : Constant  Value=-0.1
  Demux : Demux  Outputs=3
  Discrete-Time Integrator : DiscreteIntegrator  SampleTime=-1  ICPrevOutput=DiscIntNeverNeededParam  ICPrevScaledInput=DiscIntNeverNeededParam
  Homing Running Switch : Switch  Threshold=0.5
  Logical Operator1 : Logic  Operator=NOT  AllPortsSameDT=off  OutDataTypeStr=boolean
  Point-to-point trajectory : Subsystem
  Product : Product  RndMeth=Zero
  Product1 : Product  RndMeth=Zero
  Relational Operator : RelationalOperator  Operator=<=  OutDataTypeStr=boolean  RndMeth=Nearest
  Reset EncoderR : S-Function  FunctionName=ec_EboxResetEnc  Parameters=link_id, chan_id  SFunctionDeploymentMode=off  EnableBusSupport=off  mask{link_id=0, chan_id=0}
      mask prompts: link_id "Ebox ID (starting from 0)"; chan_id "Encoder channel (0 or 1)"
  Saturation : Saturate  UpperLimit=0.7  LowerLimit=-0.7
  Selector1 : Subsystem
  Stop Simulation : Stop
  Sum : Sum  Inputs=|++
  Sum1 : Sum  Inputs=|+-
  Sum2 : Sum  Inputs=|+-
  Supervisor : Stateflow chart  TreatAsAtomicUnit=on
  Terminator1 : Terminator
  Terminator2 : Terminator
  Motor R [Nm] : Outport
  airbagStatus : Outport  Port=2
  HomingBusyR : Outport  Port=3
  Ready R : Outport  Port=4
  wires:
  Homing Running Switch/1 -> AirbagSwitch/1
  Relational Operator/1 -> Supervisor/1(homeSwitch)
  Product/1 -> Saturation/1
  Point-to-point trajectory/1(ref) -> Sum/2
  Supervisor/5(homingBusy) -> Homing Running Switch/2, HomingBusyR/1
  Supervisor/3(homeControllerEnabled) -> Product/2
  Supervisor/2(toPoint) -> Point-to-point trajectory/1(toPoint)
  Supervisor/4(resetEnc) -> Reset EncoderR/1
  Logical Operator1/1 -> AirbagSwitch/2
  Supervisor/7(airBagRef) -> Sum1/1
  AirbagSwitch/1 -> Product1/1
  Product1/1 -> Motor R [Nm]/1
  Supervisor/8(controlEnabled) -> Product1/2
  Supervisor/6(airBagEnabled) -> airbagStatus/1, Logical Operator1/1
  Demux/1 -> Sum1/2, Sum2/2, Supervisor/2(carPos)
  Demux/2 -> Terminator2/1
  Selector1/1(Out1) -> Homing Running Switch/3
  controller [Nm]/1 -> Selector1/1(In1)
  carPos [m]/1 -> Demux/1, Angle2Z/1(u)
  Constant/1 -> Relational Operator/2
  Supervisor/9(Ready) -> Ready R/1
  AllReady/1 -> Supervisor/3(AllReady)
  Supervisor/10(StopSim) -> Stop Simulation/1
  Saturation/1 -> Homing Running Switch/1
  Sum2/1 -> " "/1(Input), Relational Operator/1
  " "/1(Output) -> Product/1
  Demux/3 -> Terminator1/1
  Angle2Z/1(y) -> Supervisor/4(zcoordinate)
  Sum1/1 -> "   "/1(Input)
  "   "/1(Output) -> AirbagSwitch/3
  Sum/1 -> Sum2/1
  Discrete-Time Integrator/1 -> Sum/1
  offset_homing_R/1 -> Supervisor/5(Offset_homing)
  Supervisor/1(jogSpeed) -> Discrete-Time Integrator/1

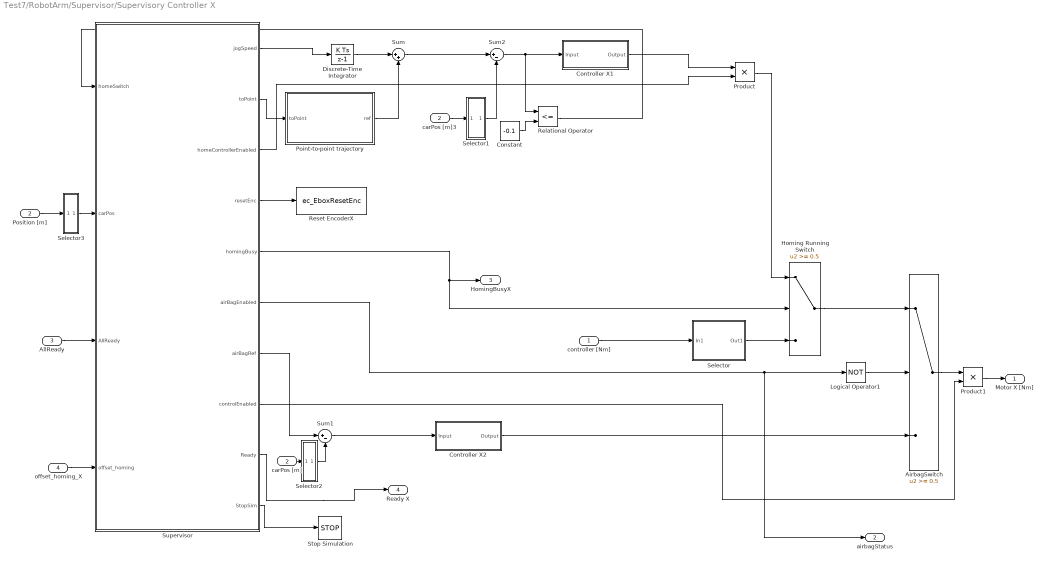
== system Test7/RobotArm/Supervisor/Supervisory Controller X ==
  controller [Nm] : Inport
  carPos [m] : Inport  Port=2
  AllReady : Inport  Port=3
  offset_homing_X : Inport  Port=4
  AirbagSwitch : Switch  Threshold=0.5
  Constant : Constant  Value=-0.1
  Controller X1 : Subsystem
  Controller X2 : Subsystem
  Discrete-Time Integrator : DiscreteIntegrator  SampleTime=-1  ICPrevOutput=DiscIntNeverNeededParam  ICPrevScaledInput=DiscIntNeverNeededParam
  Homing Running Switch : Switch  Threshold=0.5
  Logical Operator1 : Logic  Operator=NOT  AllPortsSameDT=off  OutDataTypeStr=boolean
  Point-to-point trajectory : Subsystem
  Position [m] : InportShadow  Port=2
  Product : Product  RndMeth=Zero
  Product1 : Product  RndMeth=Zero
  Relational Operator : RelationalOperator  Operator=<=  OutDataTypeStr=boolean  RndMeth=Nearest
  Reset EncoderX : S-Function  FunctionName=ec_EboxResetEnc  Parameters=link_id, chan_id  SFunctionDeploymentMode=off  EnableBusSupport=off  mask{link_id=0, chan_id=1}
      mask prompts: link_id "Ebox ID (starting from 0)"; chan_id "Encoder channel (0 or 1)"
  Selector : Subsystem
  Selector1 : Subsystem
  Selector2 : Subsystem
  Selector3 : Subsystem
  Stop Simulation : Stop
  Sum : Sum  Inputs=|++
  Sum1 : Sum  Inputs=|+-
  Sum2 : Sum  Inputs=|+-
  Supervisor : Stateflow chart  TreatAsAtomicUnit=on
  carPos [m]3 : InportShadow  Port=2
  Motor X [Nm] : Outport
  airbagStatus : Outport  Port=2
  HomingBusyX : Outport  Port=3
  Ready X : Outport  Port=4
  wires:
  Position [m]/1 -> Selector3/1(In1)
  Supervisor/6(airBagEnabled) -> airbagStatus/1, Logical Operator1/1
  Supervisor/8(controlEnabled) -> Product1/2
  Product1/1 -> Motor X [Nm]/1
  AirbagSwitch/1 -> Product1/1
  Supervisor/7(airBagRef) -> Sum1/1
  carPos [m]/1 -> Selector2/1(In1)
  Sum1/1 -> Controller X2/1(Input)
  Logical Operator1/1 -> AirbagSwitch/2
  Supervisor/4(resetEnc) -> Reset EncoderX/1
  Supervisor/2(toPoint) -> Point-to-point trajectory/1(toPoint)
  Supervisor/3(homeControllerEnabled) -> Product/2
  Supervisor/5(homingBusy) -> Homing Running Switch/2, HomingBusyX/1
  Point-to-point trajectory/1(ref) -> Sum/2
  Product/1 -> Homing Running Switch/1
  carPos [m]3/1 -> Selector1/1(In1)
  Homing Running Switch/1 -> AirbagSwitch/1
  controller [Nm]/1 -> Selector/1(In1)
  Selector/1(Out1) -> Homing Running Switch/3
  Selector1/1(Out1) -> Sum2/2
  Selector2/1(Out1) -> Sum1/2
  Relational Operator/1 -> Supervisor/1(homeSwitch)
  Constant/1 -> Relational Operator/2
  Controller X2/1(Output) -> AirbagSwitch/3
  Selector3/1(Out1) -> Supervisor/2(carPos)
  AllReady/1 -> Supervisor/3(AllReady)
  Supervisor/9(Ready) -> Ready X/1
  Supervisor/10(StopSim) -> Stop Simulation/1
  Sum2/1 -> Controller X1/1(Input), Relational Operator/1
  Controller X1/1(Output) -> Product/1
  Sum/1 -> Sum2/1
  Discrete-Time Integrator/1 -> Sum/1
  offset_homing_X/1 -> Supervisor/4(offset_homing)
  Supervisor/1(jogSpeed) -> Discrete-Time Integrator/1

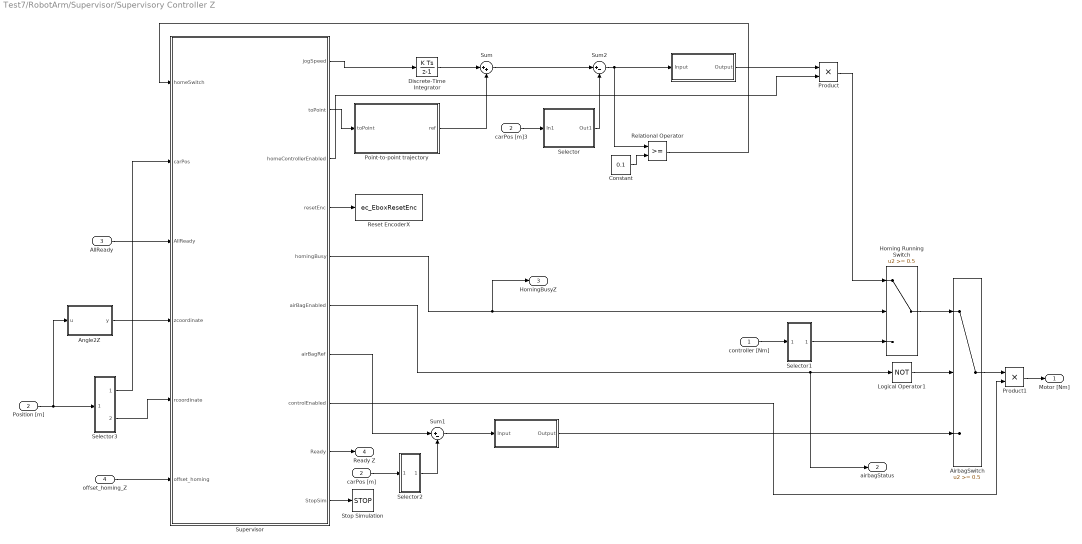
== system Test7/RobotArm/Supervisor/Supervisory Controller Z ==
  controller [Nm] : Inport
  carPos [m] : Inport  Port=2
  AllReady : Inport  Port=3
  offset_homing_Z : Inport  Port=4
  "    " : Subsystem
  "     " : Subsystem
  AirbagSwitch : Switch  Threshold=0.5
  Angle2Z : MATLAB Function  TreatAsAtomicUnit=on
  Constant : Constant  Value=0.1
  Discrete-Time Integrator : DiscreteIntegrator  SampleTime=-1  ICPrevOutput=DiscIntNeverNeededParam  ICPrevScaledInput=DiscIntNeverNeededParam
  Homing Running Switch : Switch  Threshold=0.5
  Logical Operator1 : Logic  Operator=NOT  AllPortsSameDT=off  OutDataTypeStr=boolean
  Point-to-point trajectory : Subsystem
  Position [m] : InportShadow  Port=2
  Product : Product  RndMeth=Zero
  Product1 : Product  RndMeth=Zero
  Relational Operator : RelationalOperator  OutDataTypeStr=boolean  RndMeth=Nearest
  Reset EncoderX : S-Function  FunctionName=ec_EboxResetEnc  Parameters=link_id, chan_id  SFunctionDeploymentMode=off  EnableBusSupport=off  mask{link_id=1, chan_id=0}
      mask prompts: link_id "Ebox ID (starting from 0)"; chan_id "Encoder channel (0 or 1)"
  Selector : Subsystem
  Selector1 : Subsystem
  Selector2 : Subsystem
  Selector3 : Subsystem
  Stop Simulation : Stop
  Sum : Sum  Inputs=|++
  Sum1 : Sum  Inputs=|+-
  Sum2 : Sum  Inputs=|+-
  Supervisor : Stateflow chart  TreatAsAtomicUnit=on
  carPos [m]3 : InportShadow  Port=2
  Motor [Nm] : Outport
  airbagStatus : Outport  Port=2
  HomingBusyZ : Outport  Port=3
  Ready Z : Outport  Port=4
  wires:
  Homing Running Switch/1 -> AirbagSwitch/1
  carPos [m]3/1 -> Selector/1(In1)
  controller [Nm]/1 -> Selector1/1(In1)
  Sum2/1 -> "    "/1(Input), Relational Operator/1
  Product/1 -> Homing Running Switch/1
  Point-to-point trajectory/1(ref) -> Sum/2
  Supervisor/5(homingBusy) -> Homing Running Switch/2, HomingBusyZ/1
  Supervisor/3(homeControllerEnabled) -> Product/2
  Supervisor/2(toPoint) -> Point-to-point trajectory/1(toPoint)
  Supervisor/4(resetEnc) -> Reset EncoderX/1
  Logical Operator1/1 -> AirbagSwitch/2
  Sum1/1 -> "     "/1(Input)
  carPos [m]/1 -> Selector2/1(In1)
  Supervisor/7(airBagRef) -> Sum1/1
  AirbagSwitch/1 -> Product1/1
  Product1/1 -> Motor [Nm]/1
  Supervisor/8(controlEnabled) -> Product1/2
  Supervisor/6(airBagEnabled) -> airbagStatus/1, Logical Operator1/1
  Position [m]/1 -> Angle2Z/1(u), Selector3/1(In1)
  Selector/1(Out1) -> Sum2/2
  Selector1/1(Out1) -> Homing Running Switch/3
  Selector2/1(Out1) -> Sum1/2
  Constant/1 -> Relational Operator/2
  Relational Operator/1 -> Supervisor/1(homeSwitch)
  "     "/1(Output) -> AirbagSwitch/3
  Selector3/1(Out1) -> Supervisor/2(carPos)
  AllReady/1 -> Supervisor/3(AllReady)
  Supervisor/9(Ready) -> Ready Z/1
  Supervisor/10(StopSim) -> Stop Simulation/1
  Angle2Z/1(y) -> Supervisor/4(zcoordinate)
  Selector3/2(Out2) -> Supervisor/5(rcoordinate)
  "    "/1(Output) -> Product/1
  Sum/1 -> Sum2/1
  Discrete-Time Integrator/1 -> Sum/1
  offset_homing_Z/1 -> Supervisor/6(offset_homing)
  Supervisor/1(jogSpeed) -> Discrete-Time Integrator/1

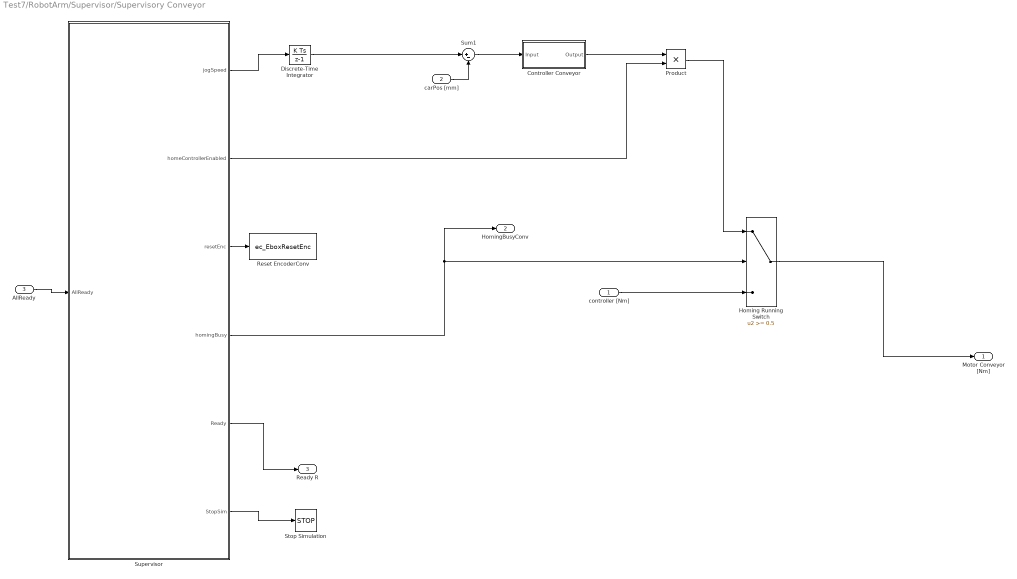
== system Test7/RobotArm/Supervisor/Supervisory Conveyor ==
  controller [Nm] : Inport
  carPos [mm] : Inport  Port=2
  AllReady : Inport  Port=3
  Controller Conveyor : Subsystem
  Discrete-Time Integrator : DiscreteIntegrator  SampleTime=-1  ICPrevOutput=DiscIntNeverNeededParam  ICPrevScaledInput=DiscIntNeverNeededParam
  Homing Running Switch : Switch  Threshold=0.5
  Product : Product  RndMeth=Zero
  Reset EncoderConv : S-Function  FunctionName=ec_EboxResetEnc  Parameters=link_id, chan_id  SFunctionDeploymentMode=off  EnableBusSupport=off  mask{link_id=1, chan_id=1}
      mask prompts: link_id "Ebox ID (starting from 0)"; chan_id "Encoder channel (0 or 1)"
  Stop Simulation : Stop
  Sum1 : Sum  Inputs=|+-
  Supervisor : Stateflow chart  TreatAsAtomicUnit=on
  Motor Conveyor [Nm] : Outport
  HomingBusyConv : Outport  Port=2
  Ready R : Outport  Port=3
  wires:
  Supervisor/1(jogSpeed) -> Discrete-Time Integrator/1
  Supervisor/4(homingBusy) -> Homing Running Switch/2, HomingBusyConv/1
  Supervisor/2(homeControllerEnabled) -> Product/2
  Supervisor/3(resetEnc) -> Reset EncoderConv/1
  Homing Running Switch/1 -> Motor Conveyor [Nm]/1
  controller [Nm]/1 -> Homing Running Switch/3
  Supervisor/5(Ready) -> Ready R/1
  AllReady/1 -> Supervisor/1(AllReady)
  Supervisor/6(StopSim) -> Stop Simulation/1
  Product/1 -> Homing Running Switch/1
  Controller Conveyor/1(Output) -> Product/1
  Discrete-Time Integrator/1 -> Sum1/1
  Sum1/1 -> Controller Conveyor/1(Input)
  carPos [mm]/1 -> Sum1/2

== system Test7/RobotArm/Supervisor/Subsystem/LED Ring ==
  U : Inport
  Subsystem : Subsystem
  Subsystem3 : Subsystem
  wires:
  U/1 -> Subsystem/1(U), Subsystem3/1(In1)
  Subsystem/1(Y) -> Subsystem3/Enable

== system Test7/RobotArm/Supervisor/Supervisory Controller R/  ==
  Input : Inport
  Dct1lowpass : sperte_lib/Dct1lowpass  f_den=100
      settings: SourceProductName=SPERTE project library
  Dctintegrator : sperte_lib/Dctintegrator  f_num=0.5
      settings: SourceProductName=SPERTE project library
  Dctleadlag : sperte_lib/Dctleadlag  f_num=6.6667  f_den=60
      settings: SourceProductName=SPERTE project library
  Gain : Gain  Gain=25
  Output : Outport
  wires:
  Input/1 -> Gain/1
  Gain/1 -> Dctintegrator/1
  Dct1lowpass/1 -> Output/1
  Dctleadlag/1 -> Dct1lowpass/1
  Dctintegrator/1 -> Dctleadlag/1

== system Test7/RobotArm/Supervisor/Supervisory Controller R/    ==
  Input : Inport
  Dct1lowpass : sperte_lib/Dct1lowpass  f_den=100
      settings: SourceProductName=SPERTE project library
  Dctleadlag : sperte_lib/Dctleadlag  f_num=6.6667  f_den=60
      settings: SourceProductName=SPERTE project library
  Gain : Gain  Gain=25
  Output : Outport
  wires:
  Gain/1 -> Dctleadlag/1
  Dctleadlag/1 -> Dct1lowpass/1
  Dct1lowpass/1 -> Output/1
  Input/1 -> Gain/1

== system Test7/RobotArm/Supervisor/Supervisory Controller R/Point-to-point trajectory ==
  toPoint : Inport
  Constant1 : Constant  Value=0
  Discrete Derivative : simulink/Discrete/Discrete Derivative  gainval=1.0  ICPrevScaledInput=0.0  OutMin=[]  OutMax=[]  OutDataType=fixdt(1, 16)  OutScaling=2^-10  DoSatur=off
  Discrete-Time Integrator : DiscreteIntegrator  InitialConditionSource=external  SampleTime=-1  ICPrevOutput=DiscIntNeverNeededParam  ICPrevScaledInput=DiscIntNeverNeededParam
  Limit Acceleration : RateLimiter  RisingSlewLimit=0.8  FallingSlewLimit=-0.8  SampleTimeMode=inherited
  Limit Speed : RateLimiter  RisingSlewLimit=0.6  FallingSlewLimit=-0.6  SampleTimeMode=inherited
  Sum : Sum  Inputs=|++
  ref : Outport
  wires:
  Sum/1 -> Limit Speed/1
  Constant1/1 -> Sum/2, Discrete-Time Integrator/2
  Limit Acceleration/1 -> Discrete-Time Integrator/1
  Discrete Derivative/1 -> Limit Acceleration/1
  Limit Speed/1 -> Discrete Derivative/1
  toPoint/1 -> Sum/1
  Discrete-Time Integrator/1 -> ref/1

== system Test7/RobotArm/Supervisor/Supervisory Controller R/Selector1 ==
  In1 : Inport
  Demux2 : Demux  Outputs=3
  Terminator4 : Terminator
  Terminator5 : Terminator
  Out1 : Outport
  wires:
  Demux2/2 -> Terminator4/1
  Demux2/3 -> Terminator5/1
  Demux2/1 -> Out1/1
  In1/1 -> Demux2/1

== system Test7/RobotArm/Supervisor/Supervisory Controller X/Controller X1 ==
  Input : Inport
  Dct1lowpass : sperte_lib/Dct1lowpass  f_den=200
      settings: SourceProductName=SPERTE project library
  Dctintegrator : sperte_lib/Dctintegrator  f_num=0.5
      settings: SourceProductName=SPERTE project library
  Dctleadlag : sperte_lib/Dctleadlag  f_num=10  f_den=90
      settings: SourceProductName=SPERTE project library
  Gain1 : Gain  Gain=20
  Output : Outport
  wires:
  Dct1lowpass/1 -> Output/1
  Dctleadlag/1 -> Dct1lowpass/1
  Input/1 -> Gain1/1
  Gain1/1 -> Dctintegrator/1
  Dctintegrator/1 -> Dctleadlag/1

== system Test7/RobotArm/Supervisor/Supervisory Controller X/Controller X2 ==
  Input : Inport
  Dct1lowpass : sperte_lib/Dct1lowpass  f_den=200
      settings: SourceProductName=SPERTE project library
  Dctleadlag : sperte_lib/Dctleadlag  f_num=10  f_den=90
      settings: SourceProductName=SPERTE project library
  Gain1 : Gain  Gain=20
  Output : Outport
  wires:
  Gain1/1 -> Dctleadlag/1
  Input/1 -> Gain1/1
  Dctleadlag/1 -> Dct1lowpass/1
  Dct1lowpass/1 -> Output/1

== system Test7/RobotArm/Supervisor/Supervisory Controller X/Point-to-point trajectory ==
  toPoint : Inport
  Constant1 : Constant  Value=0
  Discrete Derivative : simulink/Discrete/Discrete Derivative  gainval=1.0  ICPrevScaledInput=0.0  OutMin=[]  OutMax=[]  OutDataType=fixdt(1, 16)  OutScaling=2^-10  DoSatur=off
  Discrete-Time Integrator : DiscreteIntegrator  InitialConditionSource=external  SampleTime=-1  ICPrevOutput=DiscIntNeverNeededParam  ICPrevScaledInput=DiscIntNeverNeededParam
  Limit Acceleration : RateLimiter  RisingSlewLimit=0.5  FallingSlewLimit=-0.5  SampleTimeMode=inherited
  Limit Speed : RateLimiter  RisingSlewLimit=0.4  FallingSlewLimit=-0.4  SampleTimeMode=inherited
  Sum : Sum  Inputs=|++
  ref : Outport
  wires:
  Discrete-Time Integrator/1 -> ref/1
  toPoint/1 -> Sum/1
  Limit Speed/1 -> Discrete Derivative/1
  Discrete Derivative/1 -> Limit Acceleration/1
  Limit Acceleration/1 -> Discrete-Time Integrator/1
  Constant1/1 -> Discrete-Time Integrator/2, Sum/2
  Sum/1 -> Limit Speed/1

== system Test7/RobotArm/Supervisor/Supervisory Controller X/Selector ==
  In1 : Inport
  Demux2 : Demux  Outputs=3
  Terminator4 : Terminator
  Terminator5 : Terminator
  Out1 : Outport
  wires:
  Demux2/3 -> Terminator5/1
  Demux2/1 -> Terminator4/1
  In1/1 -> Demux2/1
  Demux2/2 -> Out1/1

== system Test7/RobotArm/Supervisor/Supervisory Controller X/Selector1 ==
  In1 : Inport
  Demux2 : Demux  Outputs=3
  Terminator4 : Terminator
  Terminator5 : Terminator
  Out1 : Outport
  wires:
  Demux2/2 -> Out1/1
  In1/1 -> Demux2/1
  Demux2/1 -> Terminator4/1
  Demux2/3 -> Terminator5/1

== system Test7/RobotArm/Supervisor/Supervisory Controller X/Selector2 ==
  In1 : Inport
  Demux2 : Demux  Outputs=3
  Terminator4 : Terminator
  Terminator5 : Terminator
  Out1 : Outport
  wires:
  Demux2/2 -> Out1/1
  In1/1 -> Demux2/1
  Demux2/1 -> Terminator4/1
  Demux2/3 -> Terminator5/1

== system Test7/RobotArm/Supervisor/Supervisory Controller X/Selector3 ==
  In1 : Inport
  Demux2 : Demux  Outputs=3
  Terminator4 : Terminator
  Terminator5 : Terminator
  Out1 : Outport
  wires:
  Demux2/3 -> Terminator5/1
  Demux2/1 -> Terminator4/1
  In1/1 -> Demux2/1
  Demux2/2 -> Out1/1

== system Test7/RobotArm/Supervisor/Supervisory Controller Z/     ==
  Input : Inport
  Dct1lowpass : sperte_lib/Dct1lowpass  f_den=200
      settings: SourceProductName=SPERTE project library
  Dctintegrator : sperte_lib/Dctintegrator  f_num=0.5
      settings: SourceProductName=SPERTE project library
  Dctleadlag : sperte_lib/Dctleadlag  f_num=10  f_den=90
      settings: SourceProductName=SPERTE project library
  Gain : Gain  Gain=25
  Output : Outport
  wires:
  Input/1 -> Gain/1
  Gain/1 -> Dctintegrator/1
  Dct1lowpass/1 -> Output/1
  Dctleadlag/1 -> Dct1lowpass/1
  Dctintegrator/1 -> Dctleadlag/1

== system Test7/RobotArm/Supervisor/Supervisory Controller Z/      ==
  Input : Inport
  Dct1lowpass : sperte_lib/Dct1lowpass  f_den=200
      settings: SourceProductName=SPERTE project library
  Dctleadlag : sperte_lib/Dctleadlag  f_num=10  f_den=90
      settings: SourceProductName=SPERTE project library
  Gain : Gain  Gain=30
  Output : Outport
  wires:
  Gain/1 -> Dctleadlag/1
  Dctleadlag/1 -> Dct1lowpass/1
  Dct1lowpass/1 -> Output/1
  Input/1 -> Gain/1

== system Test7/RobotArm/Supervisor/Supervisory Controller Z/Point-to-point trajectory ==
  toPoint : Inport
  Constant1 : Constant  Value=0
  Discrete Derivative : simulink/Discrete/Discrete Derivative  gainval=1.0  ICPrevScaledInput=0.0  OutMin=[]  OutMax=[]  OutDataType=fixdt(1, 16)  OutScaling=2^-10  DoSatur=off
  Discrete-Time Integrator : DiscreteIntegrator  InitialConditionSource=external  SampleTime=-1  ICPrevOutput=DiscIntNeverNeededParam  ICPrevScaledInput=DiscIntNeverNeededParam
  Limit Acceleration : RateLimiter  RisingSlewLimit=0.5  FallingSlewLimit=-0.5  SampleTimeMode=inherited
  Limit Speed : RateLimiter  RisingSlewLimit=0.2  FallingSlewLimit=-0.2  SampleTimeMode=inherited
  Sum : Sum  Inputs=|++
  ref : Outport
  wires:
  Sum/1 -> Limit Speed/1
  Constant1/1 -> Sum/2, Discrete-Time Integrator/2
  Limit Acceleration/1 -> Discrete-Time Integrator/1
  Discrete Derivative/1 -> Limit Acceleration/1
  Limit Speed/1 -> Discrete Derivative/1
  toPoint/1 -> Sum/1
  Discrete-Time Integrator/1 -> ref/1

== system Test7/RobotArm/Supervisor/Supervisory Controller Z/Selector ==
  In1 : Inport
  Demux2 : Demux  Outputs=3
  Terminator4 : Terminator
  Terminator5 : Terminator
  Out1 : Outport
  wires:
  Demux2/1 -> Terminator4/1
  In1/1 -> Demux2/1
  Demux2/2 -> Terminator5/1
  Demux2/3 -> Out1/1

== system Test7/RobotArm/Supervisor/Supervisory Controller Z/Selector1 ==
  In1 : Inport
  Demux2 : Demux  Outputs=3
  Terminator4 : Terminator
  Terminator5 : Terminator
  Out1 : Outport
  wires:
  Demux2/3 -> Out1/1
  Demux2/2 -> Terminator5/1
  In1/1 -> Demux2/1
  Demux2/1 -> Terminator4/1

== system Test7/RobotArm/Supervisor/Supervisory Controller Z/Selector2 ==
  In1 : Inport
  Demux2 : Demux  Outputs=3
  Terminator4 : Terminator
  Terminator5 : Terminator
  Out1 : Outport
  wires:
  Demux2/1 -> Terminator4/1
  In1/1 -> Demux2/1
  Demux2/2 -> Terminator5/1
  Demux2/3 -> Out1/1
